simulink model "AV"  (R2016b)
settings: Solver=ode1  StartTime=0.0  StopTime=1000000  FixedStep=0.1  RelTol=1e-3  EnableMultiTasking=on
model workspace: external: MAT-File CN.mat (data not in the file)
values from neighbouring files (symbols this model uses):
  cn0 = start_p    (= 6)    [simAV_Trace.m]
  cn1 = stop_p    (= 10)    [simAV_Trace.m]
  h = gca    [Plottrace.m]    (also in plotCells.m; plotCells_second.m)
  m = m+1    (= 1)    [plotCells.m]    (also in plotCells_second.m)
  s = [4 8 9 10 11]    [plotCells.m]    (also in plotCells_second.m)
undefined symbols (not defined in the file or in its folder): bcl, du, erp, f, hr, hs, j, pacing, r, Vh
libraries: Libs x1
settings Model: PauseTimes=18000  Creator=wai484  LastModifiedBy=wai484
settings DataIOCC: LimitDataPoints=on  SaveFormat=Array
settings OptimizationCC: LifeSpan=inf
settings DebuggingCC: SolverPrmCheckMsg=warning  SFUnexpectedBacktrackingDiag=warning  SFNoUnconditionalDefaultTransitionDiag=warning  SFExecutionAtInitializationDiag=none
settings HardwareCC: ProdBitPerPointer=32  ProdBitPerSizeT=32  ProdBitPerPtrDiffT=32  ProdLargestAtomicFloat=None  ProdIntDivRoundTo=Undefined  ProdEndianess=Unspecified  ProdWordSize=32  ProdHWDeviceType=32-bit Generic
settings ModelReferenceCC: PropagateSignalLabelsOutOfModel=off
settings GRTTargetCC: TargetLangStandard=C89/C90 (ANSI)  GeneratePreprocessorConditionals=Disable all
settings ConfigComp: CovMetricSettings=dw  CovHtmlReporting=on  CovSaveCumulativeToWorkspaceVar=on  CovSaveSingleToWorkspaceVar=on  CovExternalEMLEnable=off  CovSFcnEnable=off

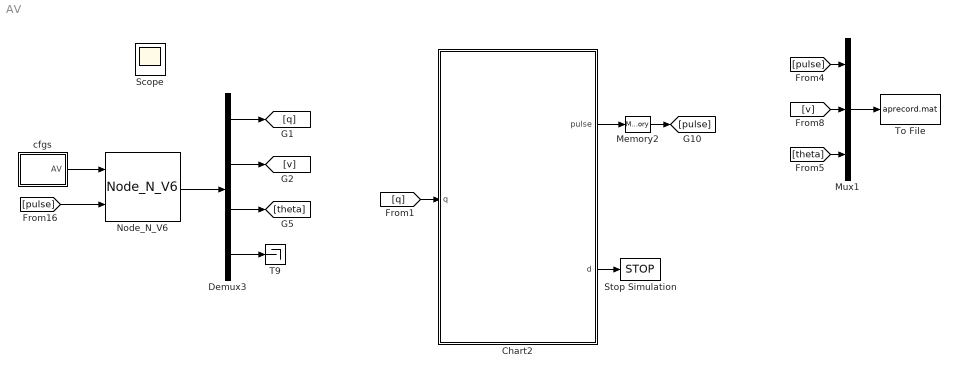
== system AV ==
  Chart2 : Stateflow chart  TreatAsAtomicUnit=on
  Demux3 : Demux  Outputs=[1, 1, 1,2]
  Memory2 : Memory
  Mux1 : Mux  Inputs=3
  Node_N_V6 : Libs/Node_N_V6
  Stop Simulation : Stop
  T9 : Terminator
  To File : ToFile  Filename=aprecord.mat  MatrixName=aprecord
      settings: Decimation=10
  cfgs : Stateflow chart  TreatAsAtomicUnit=on
  Scope : Scope
  wires:
  Node_N_V6/1 -> Demux3/1
  Mux1/1 -> To File/1
  Chart2/1(pulse) -> Memory2/1
  Demux3/4 -> T9/1
  Memory2/1 -> [pulse]
  Demux3/1 -> [q]
  Demux3/2 -> [v]
  Chart2/2(d) -> Stop Simulation/1
  Demux3/3 -> [theta]
  [pulse] -> Node_N_V6/2
  [q] -> Chart2/1(q)
  cfgs/1(AV) -> Node_N_V6/1
  [pulse] -> Mux1/1
  [theta] -> Mux1/3
  [v] -> Mux1/2

== stateflow chart AV/cfgs ==
  settings: executeAtInitialization=1
  state Ini
  (default) -> Ini : {AV=auto;}
  data: erp parameter; Vh parameter; hr parameter; hs parameter; m parameter; s parameter; j parameter; h parameter; f parameter; r parameter; bcl parameter; cfg function_output; AV output
  function cfg = auto:
    | function cfg = auto
    | 
    | BCL=bcl;
    | SD=0;
    | f1=0.1;
    | f2=0.25;
    | sigma1sq=0.0035;
    | sigma2sq=0.007;
    | 
    | d2=3.34; %av
    | erp_out=erp;
    | d0=-0.9448; %av
    | MDP=-74.65; %av
    | VT=25.05; %av
    | VR=41.25; %av
    | Vh_out=Vh;
    | 
    | hr_out=hr; 
    | hs_out=hs;
    | s_out=s;
    | j_out=j;
    | m_out=m; 
    | 
    | h_out=h;
    | f_out=f;
    | 
    | r_out=r;
    | 
    | x=135.5;
    | y=295.5;
    | 
    | cfg=[BCL, SD, f1,f2,sigma1sq, sigma2sq,d2,erp_out,d0,MDP,VT,VR,Vh_out,hr_out,hs_out,s_out,j_out,m_out,h_out,f_out,r_out,x,y];
    | 
    | end

== stateflow chart AV/Chart2 ==
  state pace
    state pace_pause [parallel]
      settings: executionOrder=1
      state q2
        du:
        t2=temporalCount (sec);
        ex:
        pp=t3+t0+t1+t2;
      state q1
        du:
        t1=temporalCount (sec);
      state q0
        du:
        t0=temporalCount (sec);
        ex:
        ERP=t2+t3+t0;
      state q3
        en: record(n,cn0,cn1,pp,ERP);
        du:
        t3=temporalCount (sec);
      (default) -> q1 : /{ n=0;t0=0;t1=0;t2=0;t3=0;}
      q1 -> q2 : [q==2]{n=n+1;}
      q0 -> q1 : [q==1]
      q2 -> q3 [order 2] : [q==3&&n==cn0 && t4<du*1000 ]/{send(start)}
      q2 -> q3 [order 1] : [q==3 && n~=cn0 && t4<du*1000 ]
      q2 -> q3 [order 4] : [q==3 && n~=-1 && t4>=du*1000 ]
      q2 -> q3 [order 3] : [q==3 && n==-1 && t4>=du*1000]/{d=1;}
      q3 -> q0 : [q==0]
    state pulseg [parallel]
      settings: executionOrder=2
      state generator
        state q01
          en:
          pulse=150;
        state q00
          en:
          pulse=0;
        (default) -> q00
        q00 -> q01 : after((pacing-10),sec)
        q01 -> q00 : after(10,sec)
      state wailt
        en:
        pulse=0;
      (default) -> wailt
      wailt -> generator : start
      generator -> wailt : di
    state Duration_t [parallel]
      settings: executionOrder=3
      state duration
        du:
        t4=temporalCount (sec);
      state Wait
      state stop
      (default) -> Wait : /{t4=0;}
      Wait -> duration : start
      duration -> stop : [t4>=du*1000 & q==3]/{send(di);n=-cn1;}
  state Idle
  (default) -> pace : {d=0; coder.extrinsic('assignin'); ERP=0; }
  pace -> Idle : [abs(d-1)<eps]
  data: nin function_input; cn0in function_input; cn1in function_input; ppin function_input; erpin function_input; pacing parameter; q input; t0 local; t2 local; t3 local; t1 local; pulse output; cn0 parameter; cn1 parameter; d output; t4 local; du parameter; ERP local; pp local; n local
  events: start local FUNCTION_CALL_EVENT; di local FUNCTION_CALL_EVENT
  function record (nin,cn0in,cn1in,ppin,erpin):
    | function record (nin,cn0in,cn1in,ppin,erpin)
    | 
    | coder.extrinsic('assignin')
    | if nin==2
    |     assignin('base', 'BCL',ppin); % Intrinsic BCL
    |     assignin('base', 'ERP0',erpin);% Intrinsic ERP
    | end
    | 
    | if nin==cn0in+11 % After the cn0 th cycle, pacing starts at the cn0+1 cycle;
    |    assignin('base', 'ERP10',erpin);% The 10th ERP 
    | end
    | 
    | if nin==-cn1in+1
    |     assignin('base', 'pause',ppin); % The maximum pause;
    |     assignin('base', 'ERPend',erpin); % The ERP when the pacing stops;
    | end
    |     
    | end
